simulink model "ProblemG_sim"  (R2022b)
settings: Solver=VariableStepAuto  StartTime=0.0  StopTime=100  RelTol=1e-3
undefined symbols (not defined in the file): A, B, C, Continuous, D, K, Time
libraries: ctrlSharedLib x1
settings Model: Creator=Pranali  LastModifiedBy=Tarun
settings SolverCC: AlgebraicLoopSolver=TrustRegion
settings DataIOCC: ReturnWorkspaceOutputs=off
settings DebuggingCC: UnconnectedInputMsg=warning  UnconnectedOutputMsg=warning  UnconnectedLineMsg=warning  SFMachineParentedDataDiag=warning  ArithmeticOperatorsInVariantConditions=warning
settings ModelReferenceCC: EnableRefExpFcnMdlSchedulingChecks=on
settings SFSimCC: CustomCodeUndefinedFunction=UseInterfaceOnly

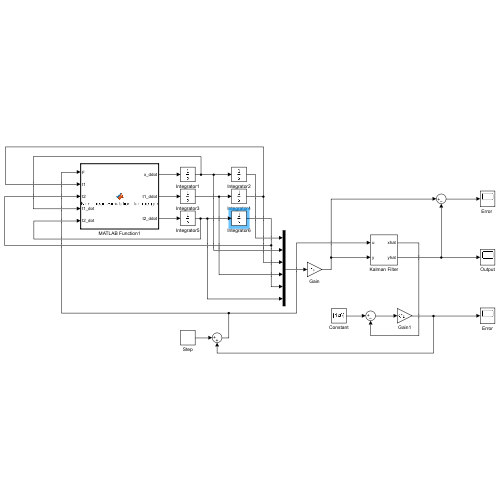
[thumbnail: Simulink's stored preview of the top-level diagram]
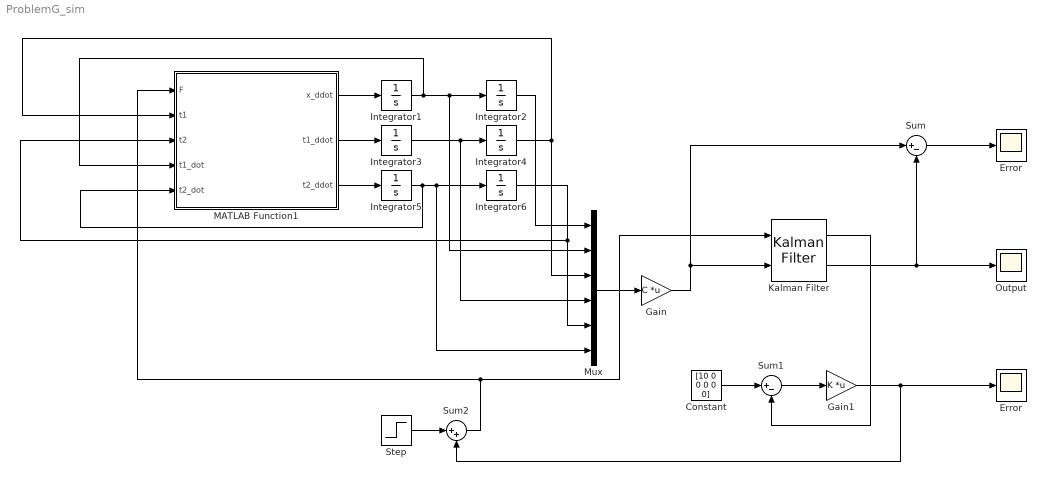
== system ProblemG_sim ==
  Constant : Constant  Value=[10 0 0 0 0 0]
  Error : Scope
  "Error " : Scope
  Gain : Gain  Gain=C  Multiplication=Matrix(K*u)
  Gain1 : Gain  Gain=K  Multiplication=Matrix(K*u)
  Integrator{1..6} (6 alike) : Integrator
  Kalman Filter : ctrlSharedLib/Kalman Filter  TimeDomain=Continuous-Time  UseCurrentEstimator=on  ModelSource=Individual A, B, C, D matrices  ModelSourceVariable=ss(A,B,C,D)  A=A  B=B  C=C  D=0  NumberOfStates=1  NumberOfInputs=1  NumberOfOutputs=1  InitialEstimateSource=Dialog  X0=[1 0 pi/6 0 pi/6 0]  P0=10  UseK=off  UseGH=off  NumberOfProcessNoiseInputs=1  G=1  TimeInvariantG=on  H=0  TimeInvariantH=on  Q=1  TimeInvariantQ=on  R=1  TimeInvariantR=on  N=0  TimeInvariantN=on  AddInputPort=on  AddEnablePort=off  OutputEstimatedY=on  OutputP=off  Ts=-1
  MATLAB Function1 : MATLAB Function  TreatAsAtomicUnit=on
  Mux : Mux  Inputs=6
  Output : Scope
  Step : Step  Time=10  SampleTime=0
  Sum : Sum  Inputs=|+-
  Sum1 : Sum  Inputs=|+-
  Sum2 : Sum  Inputs=|++
  wires:
  MATLAB Function1/2(t1_ddot) -> Integrator3/1
  Mux/1 -> Gain/1
  Step/1 -> Sum2/1
  Integrator4/1 -> MATLAB Function1/2(t1), Mux/3
  Integrator1/1 -> MATLAB Function1/4(t1_dot), Mux/2, Integrator2/1
  Integrator6/1 -> Mux/5, MATLAB Function1/3(t2)
  Gain/1 -> Sum/1, Kalman Filter/2
  Integrator3/1 -> Mux/4, Integrator4/1
  MATLAB Function1/3(t2_ddot) -> Integrator5/1
  MATLAB Function1/1(x_ddot) -> Integrator1/1
  Integrator5/1 -> MATLAB Function1/5(t2_dot), Mux/6, Integrator6/1
  Integrator2/1 -> Mux/1
  Kalman Filter/2 -> Output/1, Sum/2
  Sum/1 -> "Error "/1
  Kalman Filter/1 -> Sum1/2
  Constant/1 -> Sum1/1
  Gain1/1 -> Error/1, Sum2/2
  Sum2/1 -> Kalman Filter/1, MATLAB Function1/1(F)
  Sum1/1 -> Gain1/1

== matlab function ProblemG_sim/MATLAB Function1 ==
  data: F input; t1 input; t2 input; x_ddot output; t1_dot input; t2_dot input; t1_ddot output; t2_ddot output
function [x_ddot,t1_ddot,t2_ddot] = NonLinear_Simulation_luenberger(F,t1,t2,t1_dot,t2_dot)

%% System Parameters
l1 = 20; % length l1
l2 = 10; % length l2
m1 = 100; % mass m1
m2 = 100; % mass m2
M = 1000; % mass M
g = 9.8; % acceleration due to gravity

%% Trignometric Variables
c1 = cos(t1);
c2 = cos(t2);
s1 = sin(t1);
s2 = sin(t2);

%% x_ddot equation 
x_ddot = (F - m1*c1*s1*g - m2*c2*s2*g - m1*l1*(t1_dot^2)*(s1) - m2*l2*(t2_dot^2)*(s2))/(M + m1*(s1^2) + m2*(s2^2));

%% t1_ddot equation
t1_ddot = (x_ddot*c1 - g*s1)/l1;

%% t2_ddot equation
t2_ddot = (x_ddot*c2 - g*s2)/l2;

end
